simulink model "gm_flanger"  (R2024a)
settings: Solver=VariableStepAuto  StartTime=0.0  StopTime=20  RelTol=1e-3
settings Model: Creator=EAGLEAORUS  LastModifiedBy=fermata
settings OptimizationCC: BlockReduction=off  ConditionallyExecuteInputs=off
settings DebuggingCC: InheritedTsInSrcMsg=none

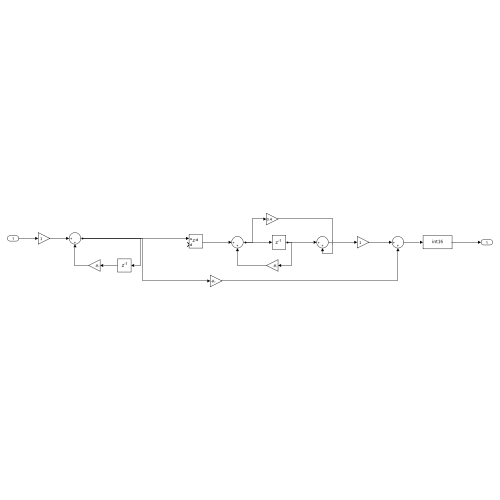
[thumbnail: Simulink's stored preview of the top-level diagram]
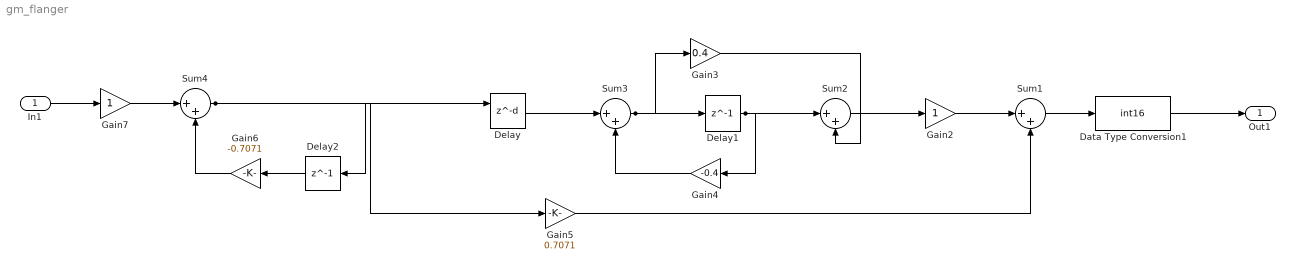
== system gm_flanger ==
  In1 : Inport  OutDataTypeStr=int16  PortDimensions=1  SampleTime=0.4
  Data Type Conversion1 : DataTypeConversion  OutDataTypeStr=int16  SaturateOnIntegerOverflow=off  RndMeth=Floor
  Delay : Delay  DelayLengthSource=Input port  DelayLength=1  DelayLengthUpperLimit=1024  InitialCondition=0  UseCircularBuffer=on
      settings: InputPortMap=u0,p1
  Delay1 : Delay  DelayLength=1  DelayLengthUpperLimit=1024  InitialCondition=0  UseCircularBuffer=on
  Delay2 : Delay  DelayLength=1  InitialCondition=0
  Gain2 : Gain  OutDataTypeStr=fixdt(1, 128, 108)
  Gain3 : Gain  Gain=0.4  OutDataTypeStr=fixdt(1, 64, 46)
  Gain4 : Gain  Gain=-0.4  OutDataTypeStr=fixdt(1, 32, 14)
  Gain5 : Gain  Gain=0.7071  OutDataTypeStr=fixdt(1, 64, 45)
  Gain6 : Gain  Gain=-0.7071  OutDataTypeStr=fixdt(1, 32, 14)
  Gain7 : Gain  OutDataTypeStr=fixdt(1, 32, 14)
  Sum1 : Sum  Inputs=|++  OutDataTypeStr=fixdt(1, 128, 108)
  Sum2 : Sum  Inputs=|++  OutDataTypeStr=fixdt(1, 64, 46)
  Sum3 : Sum  Inputs=|++  OutDataTypeStr=fixdt(1, 32, 14)
  Sum4 : Sum  Inputs=|++  OutDataTypeStr=fixdt(1, 32, 14)
  Out1 : Outport  OutDataTypeStr=int16  SampleTime=0.4
  wires:
  In1/1 -> Gain7/1
  Data Type Conversion1/1 -> Out1/1
  Delay/1 -> Sum3/1
  Delay1/1 -> Sum2/1, Gain4/1
  Delay2/1 -> Gain6/1
  Gain2/1 -> Sum1/1
  Gain3/1 -> Sum2/2
  Gain4/1 -> Sum3/2
  Gain5/1 -> Sum1/2
  Gain6/1 -> Sum4/2
  Gain7/1 -> Sum4/1
  Sum1/1 -> Data Type Conversion1/1
  Sum2/1 -> Gain2/1
  Sum3/1 -> Gain3/1, Delay1/1
  Sum4/1 -> Gain5/1, Delay2/1, Delay/1
